simulink model "larix_simulink_gazebo"  (R2020b)
settings: Solver=FixedStepDiscrete  StartTime=0.0  StopTime=inf  RelTol=1e-3  SampleTimeConstraint=Specified
values from neighbouring files (symbols this model uses):
  controller = initController(vehicle, propeller)    [init.m]
  propulsion = initPropulsion()    [init.m]
  sensors = initSensors(vehicle.pos0(3))    [init.m]
  vehicle = initVehicle()    [init.m]
undefined symbols (not defined in the file or in its folder): WMM2020
libraries: robotlib x15, sharedtransform x7, aerolibtransform2 x3, aerolibutil x3, simulink x2, aerolibatmos2 x1, aerolibgravity2 x1
settings Model: PacingRate=0.100000  Creator=pgoldschmid  LastModifiedBy=pgoldschmid

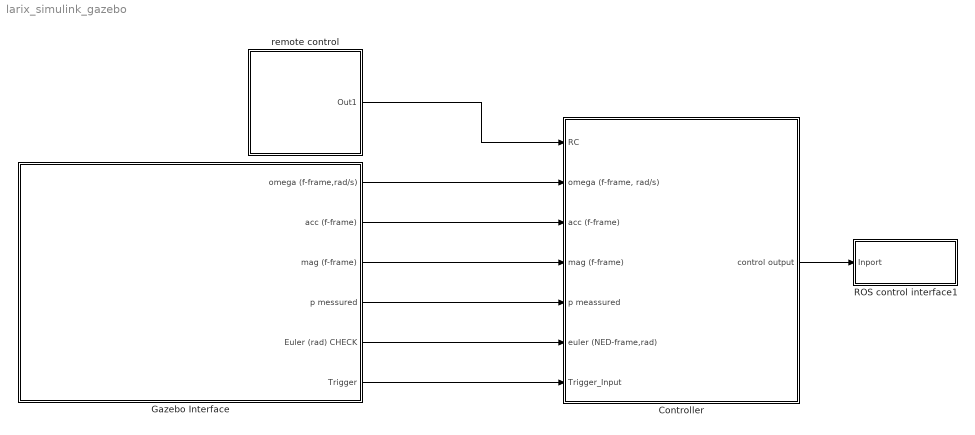
== system larix_simulink_gazebo ==
  Controller : Subsystem
      settings: PortSchema="{\"entries\":[{\"content\":{\"sides\":[{\"content\":{\"connectorIds\":[\"Out1\"]},\"type\":\"ConnectorPlacement.EquallySpacedRectSide\",\"uuid\":\"e6753237-ef8f-4a3a-b26c-e75ae99169a9\"},{\"content\":{\"connectorIds\":[\"In1\",\"In2\",\"In3\",\"In4\",\"In5\",\"In6\",\"In7\"],\"side\":\"RIGHT\"},\"type\":\"ConnectorPlacement.EquallySpacedRectSide\",\"uuid\":\"4f9edf41-85bf-437c-aaf6-18b24e8e6554\"},{\"content\":{\"connectorIds\":[],\"side\":\"TOP\"},\"type\":\"ConnectorPlacement.EquallySpacedRectSide\",\"uuid\":\"a3c7e6d1-df21-4b72-b0cf-f37c3a659b31\"},{\"content\":{\"connectorIds\":[],\"side\":\"BOTTOM\"},\"type\":\"ConnectorPlacement.EquallySpacedRectSide\",\"uuid\":\"23eac58c-75b6-4339-8a58-b1a534739bd3\"},{\"content\":{\"connectorIds\":[],\"side\":\"HIDDEN\"},\"type\":\"ConnectorPlacement.EquallySpacedRectSide\",\"uuid\":\"17e885a9-6a9e-4546-a357-6f7de688dce4\"}]},\"type\":\"ConnectorPlacement.EquallySpacedConnector\",\"uuid\":\"60ad8aaf-2408-428b-b8fd-bb77263ba152\"}],\"packageUris\":[\"http://schema.mathworks.com/mf0/Connector/R2020b\"],\"version\":\"1.0\"}"
  Gazebo Interface : Subsystem  TreatAsAtomicUnit=on
  ROS control interface1 : Subsystem  TreatAsAtomicUnit=on
  remote control : Subsystem  mask{SWA=up, SWB=up, VRA=0.0, VRB=0, SWC=up, SWD=armed (down), ThrustCmd=0.500, YawCmd=0.0, RollCmd=0.0, PitchCmd=0}
      mask prompts: SWA "Switch A"; SWB "Switch B"; VRA "tune 1 (VRA)"; VRB "tune 2 (VRB)"; SWC "Switch C"; SWD "Arming (SW D)"; ThrustCmd "Thrust Command [g]"; YawCmd "Yaw Rate Command [deg/s]"; RollCmd "Roll Command [deg]"; PitchCmd "Pitch Command [deg]"
      mask TypeOptions SWA: up | down
      mask TypeOptions SWB: up | down
      mask TypeOptions SWC: up | center | down
      mask TypeOptions SWD: disarmed (up) | armed (down)
      mask DialogControl ParameterGroupVar Prompt: Simulated Remote Control
      mask Display: image('figures/rc.jpg');
  wires:
  remote control/1(Out1) -> Controller/1(RC)
  Gazebo Interface/1(omega (f-frame,rad/s)) -> Controller/2("omega (f-frame, rad/s)")
  Gazebo Interface/2(acc (f-frame)) -> Controller/3(acc (f-frame))
  Gazebo Interface/3(mag (f-frame)) -> Controller/4(mag (f-frame))
  Gazebo Interface/4(p messured) -> Controller/5(p meassured)
  Gazebo Interface/5(Euler (rad) CHECK) -> Controller/6(euler (NED-frame,rad))
  Controller/1(control output) -> ROS control interface1/1(Inport)
  Gazebo Interface/6(Trigger) -> Controller/7(Trigger_Input)

== system larix_simulink_gazebo/Controller ==
  RC : Inport
  "omega (f-frame, rad/s)" : Inport  Port=2
  acc (f-frame) : Inport  Port=3
  mag (f-frame) : Inport  Port=4
  p meassured : Inport  Port=5
  euler (NED-frame,rad) : Inport  Port=6
  Trigger_Input : Inport  Port=7
  Triggered Subsystem : Subsystem  TreatAsAtomicUnit=on
  control output : Outport  VectorParamsAs1DForOutWhenUnconnected=off
  wires:
  Trigger_Input/1 -> Triggered Subsystem/Trigger
  Triggered Subsystem/1(control output) -> control output/1
  euler (NED-frame,rad)/1 -> Triggered Subsystem/6(euler (NED-frame,rad))
  p meassured/1 -> Triggered Subsystem/5(p meassured)
  mag (f-frame)/1 -> Triggered Subsystem/4(mag (f-frame))
  acc (f-frame)/1 -> Triggered Subsystem/3(acc (f-frame))
  RC/1 -> Triggered Subsystem/1(RC)
  "omega (f-frame, rad/s)"/1 -> Triggered Subsystem/2("omega (f-frame, rad/s)")

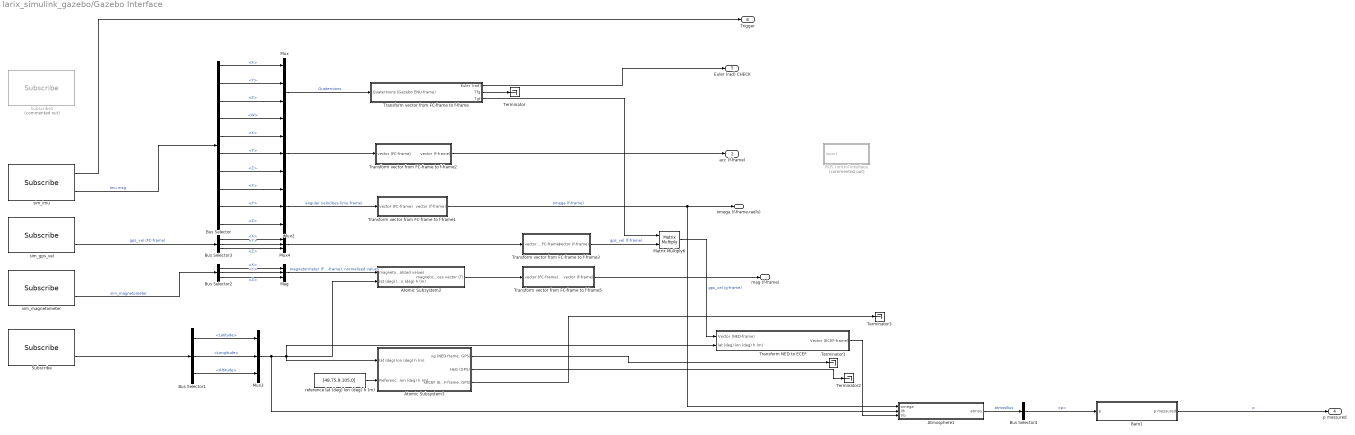
== system larix_simulink_gazebo/Gazebo Interface ==
  " " : Mux  Inputs=3
  Atmosphere1 : Subsystem
  Atomic Subsystem2 : Subsystem  TreatAsAtomicUnit=on
  Atomic Subsystem3 : Subsystem  TreatAsAtomicUnit=on
  Baro1 : Subsystem
  Bus Selector : BusSelector  OutputSignals=Orientation.X,Orientation.Y,Orientation.Z,Orientation.W,LinearAcceleration.X,LinearAcceleration.Y,LinearAcceleration.Z,AngularVelocity.X,AngularVelocity.Y,AngularVelocity.Z
  Bus Selector1 : BusSelector  OutputSignals=Latitude,Longitude,Altitude
  Bus Selector2 : BusSelector  OutputSignals=Vector.X,Vector.Y,Vector.Z
  Bus Selector3 : BusSelector  OutputSignals=Vector.X,Vector.Y,Vector.Z
  Bus Selector4 : BusSelector  OutputSignals=p
  Mag : Mux  Inputs=3
  Matrix Multiply6 : Product  Multiplication=Matrix(*)
  Mux : Mux
  Mux2 : Mux  Inputs=3
  Mux3 : Mux  Inputs=3
  Mux4 : Mux  Inputs=3
  ROS control interface : Subsystem  Commented=on  TreatAsAtomicUnit=on
  Subscribe : robotlib/Subscribe  topicSource=Select from ROS network  topic=/rrbot/sim_gps_fix  messageType=sensor_msgs/NavSatFix  SampleTime=-1  legacyBusStruct=off  messageQueueLength=1
  Subscribe1 : robotlib/Subscribe  Commented=on  topicSource=Select from ROS network  topic=/rrbot/imu_groundtruth  messageType=sensor_msgs/Imu  SampleTime=-1  legacyBusStruct=off  messageQueueLength=1
  Terminator{,1..3} (4 alike) : Terminator
  Transform NED to ECEF : Subsystem  TreatAsAtomicUnit=on
  Transform vector from FC-frame to f-frame : Subsystem  TreatAsAtomicUnit=on
  Transform vector from FC-frame to f-frame1 : Subsystem  TreatAsAtomicUnit=on
  Transform vector from FC-frame to f-frame2 : Subsystem  TreatAsAtomicUnit=on
  Transform vector from FC-frame to f-frame3 : Subsystem  TreatAsAtomicUnit=on
  Transform vector from FC-frame to f-frame5 : Subsystem  TreatAsAtomicUnit=on
  reference lat (deg) lon (deg) h (m) : Constant  Value=[48.75,9.105,0]
  sim_gps_vel : robotlib/Subscribe  topicSource=Select from ROS network  topic=/rrbot/sim_gps_vel  messageType=geometry_msgs/Vector3Stamped  SampleTime=-1  legacyBusStruct=off  messageQueueLength=1
  sim_imu : robotlib/Subscribe  topicSource=Select from ROS network  topic=/rrbot/sim_imu  messageType=sensor_msgs/Imu  SampleTime=-1  legacyBusStruct=off  messageQueueLength=1
  sim_magnetometer : robotlib/Subscribe  topicSource=Select from ROS network  topic=/rrbot/sim_magnetometer  messageType=geometry_msgs/Vector3Stamped  SampleTime=-1  legacyBusStruct=off  messageQueueLength=1
  omega (f-frame,rad/s) : Outport
  acc (f-frame) : Outport  Port=2
  mag (f-frame) : Outport  Port=3
  p messured : Outport  Port=4
  Euler (rad) CHECK : Outport  Port=5
  Trigger : Outport  Port=6
  wires:
  Bus Selector/7 -> " "/3  "<Z>"
  Bus Selector2/1 -> Mag/1  "<X>"
  Mux/1 -> Transform vector from FC-frame to f-frame/1(Quaternions (Gazebo ENU-frame))  "Quaternions"
  Mag/1 -> Atomic Subsystem2/1(magnetometer normalized values)  "magnetormeter (FC-frame), normalized values"
  Atomic Subsystem3/2(" HaG (GPS)") -> Terminator2/1
  Baro1/1(p messured) -> p messured/1  "p"
  Bus Selector/10 -> Mux2/3  "<Z>"
  Bus Selector/6 -> " "/2  "<Y>"
  Bus Selector3/2 -> Mux4/2  "<Y>"
  Bus Selector/8 -> Mux2/1  "<X>"
  Bus Selector4/1 -> Baro1/1(p)  "<p>"
  Transform vector from FC-frame to f-frame/3(Tgf) -> Matrix Multiply6/1
  Transform NED to ECEF/1(Vector (ECEF-frame)) -> Atmosphere1/3(Vb)
  sim_imu/2 -> Bus Selector/1  "Imu msg"
  Bus Selector2/3 -> Mag/3  "<Z>"
  Transform vector from FC-frame to f-frame5/1(vector (f-frame)) -> mag (f-frame)/1
  Bus Selector/3 -> Mux/3  "<Z>"
  Bus Selector2/2 -> Mag/2  "<Y>"
  Matrix Multiply6/1 -> Transform NED to ECEF/1(Vector (NED-frame))  "gps_vel (g-frame)"
  Bus Selector/5 -> " "/1  "<X>"
  Atomic Subsystem2/1(magnetic forces vector (T)) -> Transform vector from FC-frame to f-frame5/1(vector (FC-frame))
  sim_magnetometer/2 -> Bus Selector2/1  "sim_magnetometer"
  Transform vector from FC-frame to f-frame2/1(vector (f-frame)) -> acc (f-frame)/1
  Bus Selector3/3 -> Mux4/3  "<Z>"
  Bus Selector/1 -> Mux/1  "<X>"
  Mux4/1 -> Transform vector from FC-frame to f-frame3/1(vector (FC-frame))
  " "/1 -> Transform vector from FC-frame to f-frame2/1(vector (FC-frame))
  Mux2/1 -> Transform vector from FC-frame to f-frame1/1(vector (FC-frame))  "angular velocities (imu frame)"
  Atomic Subsystem3/1("xg (NED-frame, GPS)") -> Terminator1/1
  Bus Selector/2 -> Mux/2  "<Y>"
  Transform vector from FC-frame to f-frame/1(Euler (rad)) -> Euler (rad) CHECK/1
  Bus Selector/4 -> Mux/4  "<W>"
  Atmosphere1/1(atmos) -> Bus Selector4/1  "atmosBus"
  Bus Selector/9 -> Mux2/2  "<Y>"
  sim_gps_vel/2 -> Bus Selector3/1  "gps_vel (FC-frame)"
  Transform vector from FC-frame to f-frame1/1(vector (f-frame)) -> omega (f-frame,rad/s)/1, Atmosphere1/1(omega)  "omega (f-frame)"
  reference lat (deg) lon (deg) h (m)/1 -> Atomic Subsystem3/2(Reference lat (deg) lon (deg) h (m))
  Bus Selector3/1 -> Mux4/1  "<X>"
  Transform vector from FC-frame to f-frame3/1(vector (f-frame)) -> Matrix Multiply6/2  "gps_vel (f-frame)"
  Atomic Subsystem3/3("xECEF (ECEF-frame, GPS)") -> Terminator3/1
  Mux3/1 -> Atmosphere1/2(llh), Transform NED to ECEF/2(lat (deg) lon (deg) h (m)), Atomic Subsystem2/2(lat (deg) lon (deg) h (m)), Atomic Subsystem3/1(lat (deg) lon (deg) h (m))
  Bus Selector1/1 -> Mux3/1  "<Latitude>"
  Subscribe/2 -> Bus Selector1/1
  Bus Selector1/2 -> Mux3/2  "<Longitude>"
  Bus Selector1/3 -> Mux3/3  "<Altitude>"
  Transform vector from FC-frame to f-frame/2(Tfg) -> Terminator/1
  sim_imu/1 -> Trigger/1

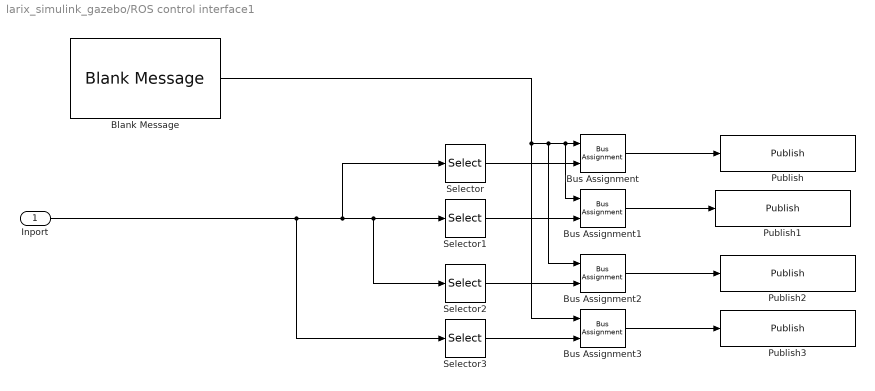
== system larix_simulink_gazebo/ROS control interface1 ==
  Inport : Inport
  Blank Message : robotlib/Blank Message  messageClass=Message  entityType=std_msgs/Float64  messageType=std_msgs/Float64  SampleTime=0.01  legacyBusStruct=off
  Bus Assignment{,1..3} (4 alike) : BusAssignment  AssignedSignals=Data
  Publish : robotlib/Publish  topicSource=Specify your own  topic=/rrbot/simulink_ros_interface/pwm/motor0  messageType=std_msgs/Float64  legacyBusStruct=off  messageQueueLength=1
  Publish1 : robotlib/Publish  topicSource=Specify your own  topic=/rrbot/simulink_ros_interface/pwm/motor1  messageType=std_msgs/Float64  legacyBusStruct=off  messageQueueLength=1
  Publish2 : robotlib/Publish  topicSource=Specify your own  topic=/rrbot/simulink_ros_interface/pwm/motor2  messageType=std_msgs/Float64  legacyBusStruct=off  messageQueueLength=1
  Publish3 : robotlib/Publish  topicSource=Specify your own  topic=/rrbot/simulink_ros_interface/pwm/motor3  messageType=std_msgs/Float64  legacyBusStruct=off  messageQueueLength=1
  Selector : Selector  InputPortWidth=4  IndexOptions=Index vector (dialog)  Indices=1  OutputSizes=1
  Selector1 : Selector  InputPortWidth=4  IndexOptions=Index vector (dialog)  Indices=2  OutputSizes=1
  Selector2 : Selector  InputPortWidth=4  IndexOptions=Index vector (dialog)  Indices=3  OutputSizes=1
  Selector3 : Selector  InputPortWidth=4  IndexOptions=Index vector (dialog)  Indices=4  OutputSizes=1
  wires:
  Inport/1 -> Selector1/1, Selector2/1, Selector/1, Selector3/1
  Selector/1 -> Bus Assignment/2
  Selector2/1 -> Bus Assignment2/2
  Bus Assignment/1 -> Publish/1
  Bus Assignment3/1 -> Publish3/1
  Blank Message/1 -> Bus Assignment/1, Bus Assignment1/1, Bus Assignment2/1, Bus Assignment3/1
  Selector1/1 -> Bus Assignment1/2
  Selector3/1 -> Bus Assignment3/2
  Bus Assignment1/1 -> Publish1/1
  Bus Assignment2/1 -> Publish2/1

== system larix_simulink_gazebo/remote control ==
  note: conversion from [g deg deg deg/s] to PWM
  note: data from mask
  note: example for automatic generation of test signals
  Bias : Bias  Bias=1500
  Bias1 : Bias  Bias=[-1 0 0 0 -1.5 -1.5 0 0 -2 -1.5]
  Bias2 : Bias  Bias=-3
  Demux : Demux  Outputs=10
  Gain : Gain  Gain=[2, 1/45, 1/45, 1/90, 4 4 2 2 2 4]*500
  Mux : Mux  Inputs=10
  Pulse Generator : DiscretePulseGenerator  PulseType=Time based  Amplitude=6  Period=10  PulseWidth=50
  rc : Constant  Value=[ThrustCmd RollCmd PitchCmd YawCmd SWA SWB VRA VRB SWC SWD]
  test signal switch : ManualSwitch
  Out1 : Outport  VectorParamsAs1DForOutWhenUnconnected=off
  wires:
  Demux/10 -> Mux/10
  Demux/9 -> Mux/9
  Demux/8 -> Mux/8
  Demux/7 -> Mux/7
  Demux/6 -> Mux/6
  Demux/5 -> Mux/5
  Demux/2 -> test signal switch/1
  Bias2/1 -> test signal switch/2
  test signal switch/1 -> Mux/2
  Pulse Generator/1 -> Bias2/1
  Mux/1 -> Bias1/1
  rc/1 -> Demux/1
  Demux/4 -> Mux/4
  Demux/3 -> Mux/3
  Demux/1 -> Mux/1
  Bias1/1 -> Gain/1
  Bias/1 -> Out1/1
  Gain/1 -> Bias/1

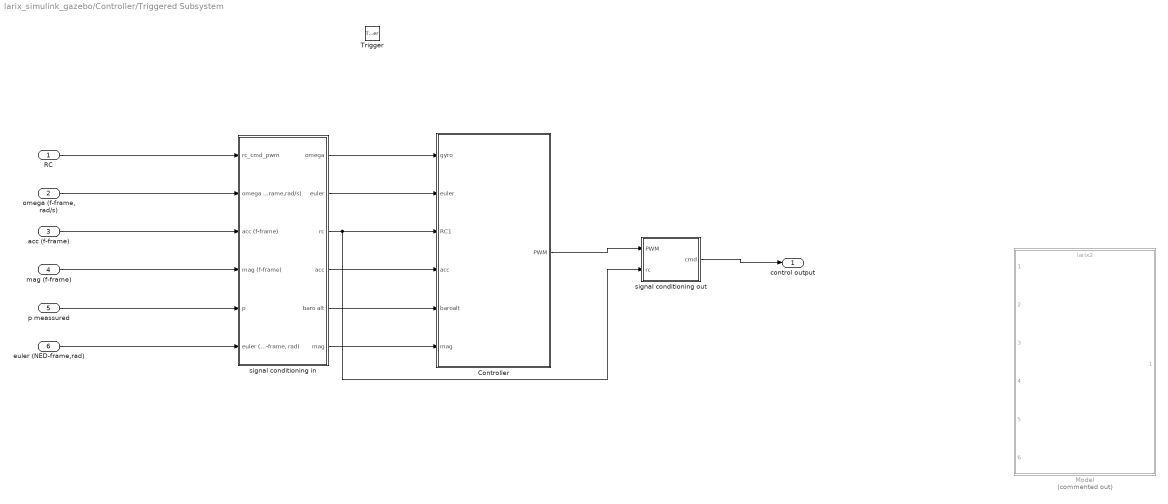
== system larix_simulink_gazebo/Controller/Triggered Subsystem ==
  RC : Inport
  "omega (f-frame, rad/s)" : Inport  Port=2
  acc (f-frame) : Inport  Port=3
  mag (f-frame) : Inport  Port=4
  p meassured : Inport  Port=5
  euler (NED-frame,rad) : Inport  Port=6
  Trigger : TriggerPort  VariantControl=Variant
  Controller : Subsystem  TreatAsAtomicUnit=on
  Model : ModelReference  Commented=on  ModelNameDialog=larix2.slx  SimulationMode=Normal  ModelReferenceVersion=5.6
  signal conditioning in : Subsystem
  signal conditioning out : Subsystem
  control output : Outport
  wires:
  signal conditioning out/1(cmd) -> control output/1
  signal conditioning in/5(baro alt) -> Controller/5(baroalt)
  signal conditioning in/3(rc) -> Controller/3(RC1), signal conditioning out/2(rc)
  signal conditioning in/4(acc) -> Controller/4(acc)
  "omega (f-frame, rad/s)"/1 -> signal conditioning in/2(omega (f-frame,rad/s))
  acc (f-frame)/1 -> signal conditioning in/3(acc (f-frame))
  signal conditioning in/2(euler) -> Controller/2(euler)
  euler (NED-frame,rad)/1 -> signal conditioning in/6("euler (NED-frame, rad)")
  signal conditioning in/1(omega) -> Controller/1(gyro)
  signal conditioning in/6(mag) -> Controller/6(mag)
  RC/1 -> signal conditioning in/1(rc_cmd_pwm)
  mag (f-frame)/1 -> signal conditioning in/4(mag (f-frame))
  p meassured/1 -> signal conditioning in/5(p)
  Controller/1(PWM) -> signal conditioning out/1(PWM)

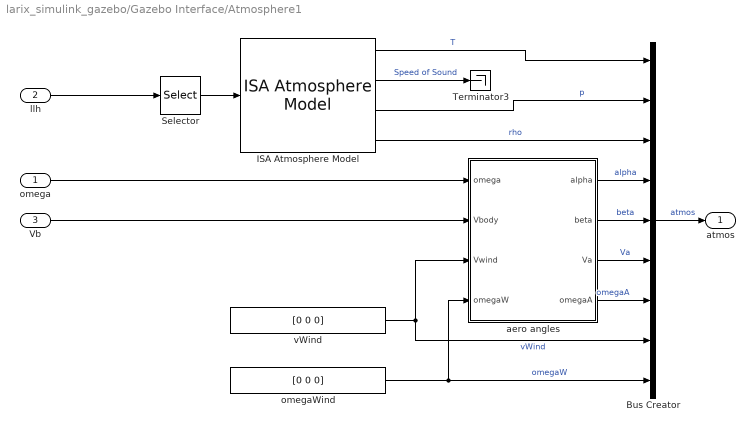
== system larix_simulink_gazebo/Gazebo Interface/Atmosphere1 ==
  omega : Inport
  llh : Inport  Port=2
  Vb : Inport  Port=3
  Bus Creator : BusCreator  Inputs=9
  ISA Atmosphere Model : aerolibatmos2/ISA Atmosphere Model  custom=off  g=9.80665  gamma=1.4  R=287.0531  L=0.0065  h_trop=11000  h_strat=20000  rho0=1.225  P0=101325  T0=288.15  h0=0
  Selector : Selector  InputPortWidth=3  IndexOptions=Index vector (dialog)  Indices=3  OutputSizes=1
  Terminator3 : Terminator
  aero angles : MATLAB Function  TreatAsAtomicUnit=on
  omegaWind : Constant  Value=[0 0 0]  SampleTime=-1
  vWind : Constant  Value=[0 0 0]  SampleTime=-1
  atmos : Outport  VectorParamsAs1DForOutWhenUnconnected=off
  wires:
  vWind/1 -> Bus Creator/8, aero angles/3(Vwind)  "vWind"
  omegaWind/1 -> Bus Creator/9, aero angles/4(omegaW)  "omegaW"
  aero angles/4(omegaA) -> Bus Creator/7  "omegaA"
  Vb/1 -> aero angles/2(Vbody)
  omega/1 -> aero angles/1(omega)
  aero angles/2(beta) -> Bus Creator/5  "beta"
  aero angles/1(alpha) -> Bus Creator/4  "alpha"
  aero angles/3(Va) -> Bus Creator/6  "Va"
  ISA Atmosphere Model/4 -> Bus Creator/3  "rho"
  Selector/1 -> ISA Atmosphere Model/1
  llh/1 -> Selector/1
  ISA Atmosphere Model/2 -> Terminator3/1  "Speed of Sound"
  ISA Atmosphere Model/1 -> Bus Creator/1  "T"
  ISA Atmosphere Model/3 -> Bus Creator/2  "p"
  Bus Creator/1 -> atmos/1  "atmos"

== system larix_simulink_gazebo/Gazebo Interface/Atomic Subsystem2 ==
  magnetometer normalized values : Inport
  lat (deg) lon (deg) h (m) : Inport  Port=2
  Demux : Demux  Outputs=3
  Gain : Gain  Gain=0.000000001
  Product : Product
  World Magnetic Model : aerolibgravity2/World Magnetic Model  model=WMM2020 (2020-2025)  customFile='WMM2020.COF'  units=Metric (MKS)  time_in=off  month=October  day=25  year=2021  action=Error  h_out=off  dec_out=off  inc_out=off  ti_out=on
      settings: SourceProductBaseCode=AE
  magnetic forces vector (T) : Outport
  wires:
  Product/1 -> magnetic forces vector (T)/1
  Gain/1 -> Product/2  "Intensity of magnetic force (T)"
  magnetometer normalized values/1 -> Product/1
  World Magnetic Model/2 -> Gain/1  "Intensity of magnetic force"
  Demux/3 -> World Magnetic Model/1
  Demux/1 -> World Magnetic Model/2
  Demux/2 -> World Magnetic Model/3
  lat (deg) lon (deg) h (m)/1 -> Demux/1

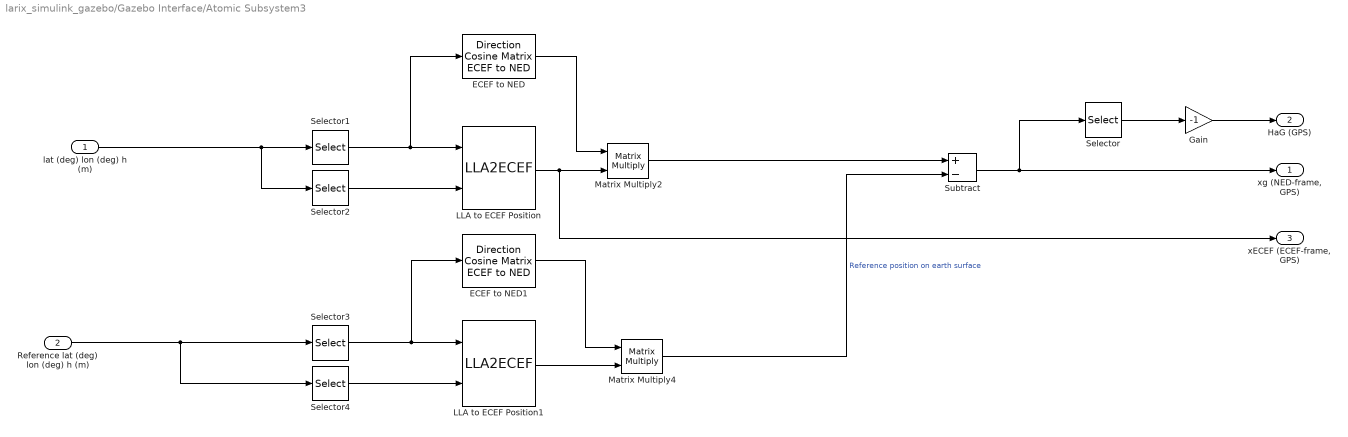
== system larix_simulink_gazebo/Gazebo Interface/Atomic Subsystem3 ==
  lat (deg) lon (deg) h (m) : Inport
  Reference lat (deg) lon (deg) h (m) : Inport  Port=2
  ECEF to NED : aerolibtransform2/Direction Cosine Matrix ECEF to NED
      settings: SourceProductBaseCode=AE
  ECEF to NED1 : aerolibtransform2/Direction Cosine Matrix ECEF to NED
      settings: SourceProductBaseCode=AE
  Gain : Gain  Gain=-1
  LLA to ECEF Position : LLA2ECEF
  LLA to ECEF Position1 : LLA2ECEF
  Matrix Multiply2 : Product  Multiplication=Matrix(*)
  Matrix Multiply4 : Product  Multiplication=Matrix(*)
  Selector : Selector  InputPortWidth=3  IndexOptions=Index vector (dialog)  Indices=[3]  OutputSizes=1
  Selector1 : Selector  InputPortWidth=3  IndexOptions=Index vector (dialog)  Indices=[1 2]  OutputSizes=1
  Selector2 : Selector  InputPortWidth=3  IndexOptions=Index vector (dialog)  Indices=[3]  OutputSizes=1
  Selector3 : Selector  InputPortWidth=3  IndexOptions=Index vector (dialog)  Indices=[1 2]  OutputSizes=1
  Selector4 : Selector  InputPortWidth=3  IndexOptions=Index vector (dialog)  Indices=[3]  OutputSizes=1
  Subtract : Sum  Inputs=+-
  "xg (NED-frame, GPS)" : Outport
  " HaG (GPS)" : Outport  Port=2
  "xECEF (ECEF-frame, GPS)" : Outport  Port=3
  wires:
  ECEF to NED1/1 -> Matrix Multiply4/1
  LLA to ECEF Position1/1 -> Matrix Multiply4/2
  Matrix Multiply4/1 -> Subtract/2  "Reference position on earth surface"
  LLA to ECEF Position/1 -> "xECEF (ECEF-frame, GPS)"/1, Matrix Multiply2/2
  lat (deg) lon (deg) h (m)/1 -> Selector2/1, Selector1/1
  Selector1/1 -> ECEF to NED/1, LLA to ECEF Position/1
  Selector2/1 -> LLA to ECEF Position/2
  ECEF to NED/1 -> Matrix Multiply2/1
  Matrix Multiply2/1 -> Subtract/1
  Reference lat (deg) lon (deg) h (m)/1 -> Selector4/1, Selector3/1
  Selector4/1 -> LLA to ECEF Position1/2
  Selector3/1 -> ECEF to NED1/1, LLA to ECEF Position1/1
  Subtract/1 -> Selector/1, "xg (NED-frame, GPS)"/1
  Selector/1 -> Gain/1
  Gain/1 -> " HaG (GPS)"/1

== system larix_simulink_gazebo/Gazebo Interface/Baro1 ==
  p : Inport  PortDimensions=1
  Baro Bias : Constant  Value=sensors.Baro.Bias
  Baro Noise : RandomNumber  Variance=sensors.Baro.Noise^2
  Manual Switch2 : ManualSwitch
  Sum3 : Sum  Inputs=++|
  Sum4 : Sum  Inputs=++|
  p messured : Outport  PortDimensions=1  VectorParamsAs1DForOutWhenUnconnected=off
  wires:
  Sum3/1 -> Sum4/2
  Sum4/1 -> Manual Switch2/1
  Manual Switch2/1 -> p messured/1
  p/1 -> Manual Switch2/2, Sum3/2  "p [Pa]"
  Baro Bias/1 -> Sum4/1
  Baro Noise/1 -> Sum3/1

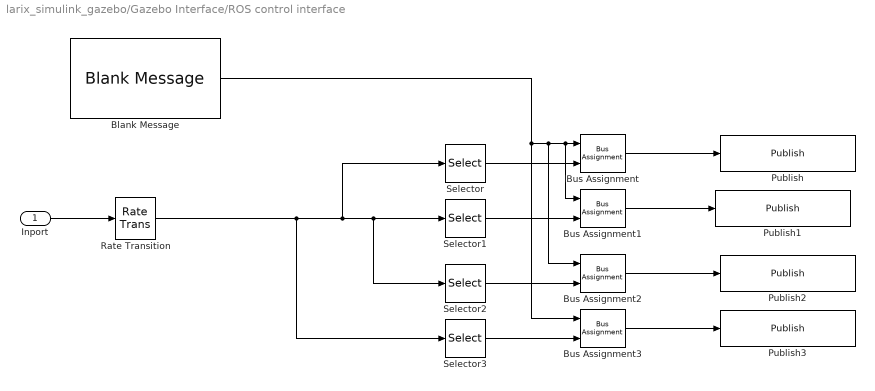
== system larix_simulink_gazebo/Gazebo Interface/ROS control interface ==
  Inport : Inport
  Blank Message : robotlib/Blank Message  messageClass=Message  entityType=std_msgs/Float64  messageType=std_msgs/Float64  SampleTime=0.01  legacyBusStruct=off
  Bus Assignment{,1..3} (4 alike) : BusAssignment  AssignedSignals=Data
  Publish : robotlib/Publish  topicSource=Specify your own  topic=/rrbot/simulink_ros_interface/pwm/motor0  messageType=std_msgs/Float64  legacyBusStruct=off  messageQueueLength=1
  Publish1 : robotlib/Publish  topicSource=Specify your own  topic=/rrbot/simulink_ros_interface/pwm/motor1  messageType=std_msgs/Float64  legacyBusStruct=off  messageQueueLength=1
  Publish2 : robotlib/Publish  topicSource=Specify your own  topic=/rrbot/simulink_ros_interface/pwm/motor2  messageType=std_msgs/Float64  legacyBusStruct=off  messageQueueLength=1
  Publish3 : robotlib/Publish  topicSource=Specify your own  topic=/rrbot/simulink_ros_interface/pwm/motor3  messageType=std_msgs/Float64  legacyBusStruct=off  messageQueueLength=1
  Rate Transition : RateTransition  OutPortSampleTime=0.01
  Selector : Selector  InputPortWidth=4  IndexOptions=Index vector (dialog)  Indices=3  OutputSizes=1
  Selector1 : Selector  InputPortWidth=4  IndexOptions=Index vector (dialog)  Indices=4  OutputSizes=1
  Selector2 : Selector  InputPortWidth=4  IndexOptions=Index vector (dialog)  Indices=2  OutputSizes=1
  Selector3 : Selector  InputPortWidth=4  IndexOptions=Index vector (dialog)  Indices=1  OutputSizes=1
  wires:
  Bus Assignment2/1 -> Publish2/1
  Bus Assignment1/1 -> Publish1/1
  Selector3/1 -> Bus Assignment3/2
  Selector1/1 -> Bus Assignment1/2
  Blank Message/1 -> Bus Assignment3/1, Bus Assignment2/1, Bus Assignment1/1, Bus Assignment/1
  Bus Assignment3/1 -> Publish3/1
  Bus Assignment/1 -> Publish/1
  Selector2/1 -> Bus Assignment2/2
  Selector/1 -> Bus Assignment/2
  Inport/1 -> Rate Transition/1
  Rate Transition/1 -> Selector3/1, Selector/1, Selector2/1, Selector1/1

== system larix_simulink_gazebo/Gazebo Interface/Transform NED to ECEF ==
  Vector (NED-frame) : Inport
  lat (deg) lon (deg) h (m) : Inport  Port=2
  ECEF to NED : aerolibtransform2/Direction Cosine Matrix ECEF to NED
      settings: SourceProductBaseCode=AE
  Matrix Multiply7 : Product  Multiplication=Matrix(*)
  NED to ECEF : aerolibutil/Invert  3x3 Matrix
  Selector1 : Selector  InputPortWidth=3  IndexOptions=Index vector (dialog)  Indices=[1 2]  OutputSizes=1
  Vector (ECEF-frame) : Outport
  wires:
  Selector1/1 -> ECEF to NED/1
  lat (deg) lon (deg) h (m)/1 -> Selector1/1
  NED to ECEF/1 -> Matrix Multiply7/1
  ECEF to NED/1 -> NED to ECEF/1
  Vector (NED-frame)/1 -> Matrix Multiply7/2
  Matrix Multiply7/1 -> Vector (ECEF-frame)/1  "gps_vel (ecef-frame)"

== system larix_simulink_gazebo/Gazebo Interface/Transform vector from FC-frame to f-frame ==
  Quaternions (Gazebo ENU-frame) : Inport
  Quaternions to Tfg : sharedtransform/Quaternions to  Direction Cosine Matrix  aMode=aMode
      settings: SourceProductBaseCode=AE,PW,MT,UV,VE,VP
  Reorder to phi theta psi : Selector  InputPortWidth=3  IndexOptions=Index vector (dialog)  Indices=[3,2,1]  OutputSizes=1
  Rotation angles : sharedtransform/Quaternions to Rotation Angles  rotationOrder=ZYX  aMode=aMode
      settings: SourceProductBaseCode=AE,PW,MT,UV,VE,VP
  Tgf1 : aerolibutil/Invert  3x3 Matrix
  Transform Gazebo ENU-frame to NED-frame : Subsystem  TreatAsAtomicUnit=on
  Euler (rad) : Outport
  Tfg : Outport  Port=2
  Tgf : Outport  Port=3
  wires:
  Reorder to phi theta psi/1 -> Euler (rad)/1
  Quaternions to Tfg/1 -> Tfg/1, Tgf1/1
  Transform Gazebo ENU-frame to NED-frame/1(Quaternion (NED-frame)) -> Rotation angles/1, Quaternions to Tfg/1
  Rotation angles/1 -> Reorder to phi theta psi/1
  Tgf1/1 -> Tgf/1
  Quaternions (Gazebo ENU-frame)/1 -> Transform Gazebo ENU-frame to NED-frame/1("Quaternion (ENU-frame, Gazebo reference)")

== system larix_simulink_gazebo/Gazebo Interface/Transform vector from FC-frame to f-frame1 ==
  vector (FC-frame) : Inport
  Matrix Multiply1 : Product  Multiplication=Matrix(*)
  Rotation angles of FC-frame wrt f-frame : Constant  Value=[3.141592,0,0]
  T_f_FC : sharedtransform/Rotation Angles to Direction Cosine Matrix  rotationOrder=XYZ  aMode=aMode
      settings: SourceProductBaseCode=AE,PW,MT,UV,VE,VP
  vector (f-frame) : Outport
  wires:
  vector (FC-frame)/1 -> Matrix Multiply1/2  "input vector (FC-frame)"
  Matrix Multiply1/1 -> vector (f-frame)/1  "output vector (f-frame)"
  Rotation angles of FC-frame wrt f-frame/1 -> T_f_FC/1
  T_f_FC/1 -> Matrix Multiply1/1

== system larix_simulink_gazebo/Gazebo Interface/Transform vector from FC-frame to f-frame2 ==
  vector (FC-frame) : Inport
  Matrix Multiply1 : Product  Multiplication=Matrix(*)
  Rotation angles of FC-frame wrt f-frame : Constant  Value=[3.141592,0,0]
  T_f_FC : sharedtransform/Rotation Angles to Direction Cosine Matrix  rotationOrder=XYZ  aMode=aMode
      settings: SourceProductBaseCode=AE,PW,MT,UV,VE,VP
  vector (f-frame) : Outport
  wires:
  vector (FC-frame)/1 -> Matrix Multiply1/2  "input vector (FC-frame)"
  Matrix Multiply1/1 -> vector (f-frame)/1  "output vector (f-frame)"
  Rotation angles of FC-frame wrt f-frame/1 -> T_f_FC/1
  T_f_FC/1 -> Matrix Multiply1/1

== system larix_simulink_gazebo/Gazebo Interface/Transform vector from FC-frame to f-frame3 ==
  vector (FC-frame) : Inport
  Matrix Multiply1 : Product  Multiplication=Matrix(*)
  Rotation angles of FC-frame wrt f-frame : Constant  Value=[3.141592,0,0]
  T_f_FC : sharedtransform/Rotation Angles to Direction Cosine Matrix  rotationOrder=XYZ  aMode=aMode
      settings: SourceProductBaseCode=AE,PW,MT,UV,VE,VP
  vector (f-frame) : Outport
  wires:
  vector (FC-frame)/1 -> Matrix Multiply1/2  "input vector (FC-frame)"
  Matrix Multiply1/1 -> vector (f-frame)/1  "output vector (f-frame)"
  Rotation angles of FC-frame wrt f-frame/1 -> T_f_FC/1
  T_f_FC/1 -> Matrix Multiply1/1

== system larix_simulink_gazebo/Gazebo Interface/Transform vector from FC-frame to f-frame5 ==
  vector (FC-frame) : Inport
  Matrix Multiply1 : Product  Multiplication=Matrix(*)
  Rotation angles of FC-frame wrt f-frame : Constant  Value=[3.141592,0,0]
  T_f_FC : sharedtransform/Rotation Angles to Direction Cosine Matrix  rotationOrder=XYZ  aMode=aMode
      settings: SourceProductBaseCode=AE,PW,MT,UV,VE,VP
  vector (f-frame) : Outport
  wires:
  vector (FC-frame)/1 -> Matrix Multiply1/2  "input vector (FC-frame)"
  Matrix Multiply1/1 -> vector (f-frame)/1  "output vector (f-frame)"
  Rotation angles of FC-frame wrt f-frame/1 -> T_f_FC/1
  T_f_FC/1 -> Matrix Multiply1/1

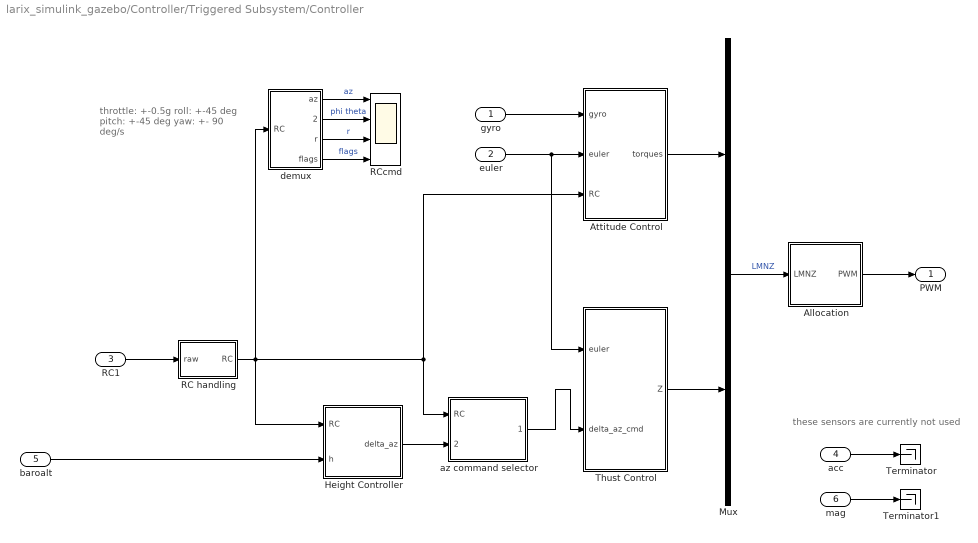
== system larix_simulink_gazebo/Controller/Triggered Subsystem/Controller ==
  note: these sensors are currently not used
  note: throttle: +-0.5g
      | roll: +-45 deg
      | pitch: +-45 deg
      | yaw: +- 90 deg/s
  gyro : Inport  OutDataTypeStr=single  PortDimensions=3
  euler : Inport  Port=2  OutDataTypeStr=single  PortDimensions=3
  RC1 : Inport  Port=3  OutDataTypeStr=single  PortDimensions=10
  acc : Inport  Port=4  OutDataTypeStr=single  PortDimensions=3
  baroalt : Inport  Port=5  OutDataTypeStr=single  PortDimensions=1
  mag : Inport  Port=6  OutDataTypeStr=single  PortDimensions=3
  Allocation : Subsystem
  Attitude Control : Subsystem
  Height Controller : Subsystem
  Mux : Mux  Inputs=2
  RC handling : Subsystem
  RCcmd : Scope  NumInputPorts=4
  Terminator : Terminator
  Terminator1 : Terminator
  Thust Control : Subsystem
  az command selector : Subsystem
  demux : Subsystem
  PWM : Outport  OutDataTypeStr=single  PortDimensions=4  VectorParamsAs1DForOutWhenUnconnected=off
  wires:
  Height Controller/1(delta_az) -> az command selector/2(az_hctrl)
  RC1/1 -> RC handling/1(raw)
  Mux/1 -> Allocation/1(LMNZ)  "LMNZ"
  mag/1 -> Terminator1/1
  demux/3(r) -> RCcmd/3  "r"
  demux/1(az) -> RCcmd/1  "az"
  az command selector/1(az_cmd) -> Thust Control/2(delta_az_cmd)
  Attitude Control/1(torques) -> Mux/1
  baroalt/1 -> Height Controller/2(h)
  demux/2(phitheta) -> RCcmd/2  "phi theta"
  acc/1 -> Terminator/1
  demux/4(flags) -> RCcmd/4  "flags"
  euler/1 -> Thust Control/1(euler), Attitude Control/2(euler)
  Thust Control/1(Z) -> Mux/2
  gyro/1 -> Attitude Control/1(gyro)
  RC handling/1(RC) -> az command selector/1(RC), Attitude Control/3(RC), Height Controller/1(RC), demux/1(RC)
  Allocation/1(PWM) -> PWM/1

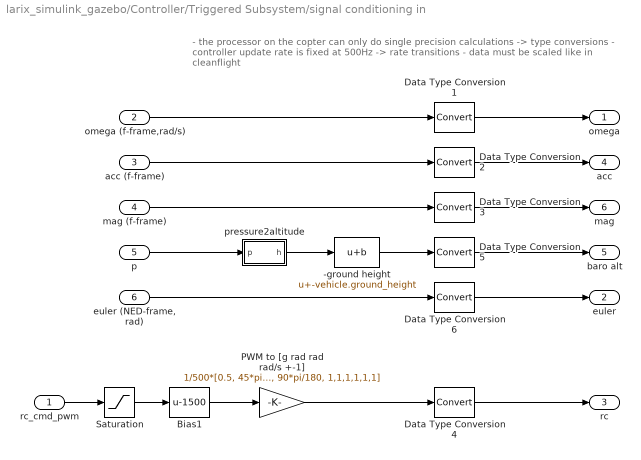
== system larix_simulink_gazebo/Controller/Triggered Subsystem/signal conditioning in ==
  note: - the processor on the copter can only do single precision calculations -> type conversions
      | - controller update rate is fixed at 500Hz -> rate transitions
      | - data must be scaled like in cleanflight
  rc_cmd_pwm : Inport  PortDimensions=10
  omega (f-frame,rad/s) : Inport  Port=2
  acc (f-frame) : Inport  Port=3
  mag (f-frame) : Inport  Port=4
  p : Inport  Port=5
  "euler (NED-frame, rad)" : Inport  Port=6
  -ground height : Bias  Bias=-vehicle.ground_height
  Bias1 : Bias  Bias=-1500
  Data Type Conversion{1..6} (6 alike) : DataTypeConversion
  PWM to [g rad rad rad/s +-1] : Gain  Gain=1/500*[0.5, 45*pi/180, 45*pi/180, 90*pi/180, 1,1,1,1,1,1]
  Saturation : Saturate  UpperLimit=2000  LowerLimit=1000
  pressure2altitude : MATLAB Function  TreatAsAtomicUnit=on
  omega : Outport  VectorParamsAs1DForOutWhenUnconnected=off
  euler : Outport  Port=2  PortDimensions=3  VectorParamsAs1DForOutWhenUnconnected=off
  rc : Outport  Port=3  VectorParamsAs1DForOutWhenUnconnected=off
  acc : Outport  Port=4  VectorParamsAs1DForOutWhenUnconnected=off
  baro alt : Outport  Port=5  VectorParamsAs1DForOutWhenUnconnected=off
  mag : Outport  Port=6  VectorParamsAs1DForOutWhenUnconnected=off
  wires:
  "euler (NED-frame, rad)"/1 -> Data Type Conversion6/1
  omega (f-frame,rad/s)/1 -> Data Type Conversion1/1
  PWM to [g rad rad rad/s +-1]/1 -> Data Type Conversion4/1
  Bias1/1 -> PWM to [g rad rad rad/s +-1]/1
  Data Type Conversion6/1 -> euler/1
  Saturation/1 -> Bias1/1
  rc_cmd_pwm/1 -> Saturation/1
  Data Type Conversion4/1 -> rc/1
  Data Type Conversion5/1 -> baro alt/1
  Data Type Conversion3/1 -> mag/1
  Data Type Conversion2/1 -> acc/1
  Data Type Conversion1/1 -> omega/1
  mag (f-frame)/1 -> Data Type Conversion3/1
  acc (f-frame)/1 -> Data Type Conversion2/1
  p/1 -> pressure2altitude/1(p)
  -ground height/1 -> Data Type Conversion5/1
  pressure2altitude/1(h) -> -ground height/1

== system larix_simulink_gazebo/Controller/Triggered Subsystem/signal conditioning out ==
  note: this simulates the arming handling
      | inside the onboard computer
      | (engines off if switch off)
  PWM : Inport
  rc : Inport  Port=2
  Compare To Constant : simulink/Logic and Bit Operations/Compare To Constant  relop=>  const=0  OutDataTypeStr=boolean
  Data Type Conversion1 : DataTypeConversion
  Delay2 : Delay  DelayLength=1
  Selector : Selector  IndexMode=Zero-based  InputPortWidth=10  IndexOptions=Index vector (dialog)  Indices=9  OutputSizes=1
  Switch : Switch  Criteria=u2 > Threshold
  motors off : Constant  Value=1000.*ones(4,1)
  cmd : Outport  VectorParamsAs1DForOutWhenUnconnected=off
  wires:
  rc/1 -> Selector/1
  motors off/1 -> Switch/3
  Delay2/1 -> Switch/1
  Switch/1 -> cmd/1
  Compare To Constant/1 -> Switch/2
  Selector/1 -> Compare To Constant/1
  Data Type Conversion1/1 -> Delay2/1
  PWM/1 -> Data Type Conversion1/1

== system larix_simulink_gazebo/Gazebo Interface/Transform vector from FC-frame to f-frame/Transform Gazebo ENU-frame to NED-frame ==
  "Quaternion (ENU-frame, Gazebo reference)" : Inport
  Constant : Constant  Value=[0,0,pi/2]
  Gain : Gain  Gain=[1,1,-1,-1]
  Quaternion Multiplication : aerolibutil/Quaternion Multiplication
  Reorder real part : Selector  InputPortWidth=4  IndexOptions=Index vector (dialog)  Indices=[4,1,2,3]  OutputSizes=1
  Rotation Angles to Quaternions : sharedtransform/Rotation Angles to Quaternions  rotationOrder=XYZ  aMode=aMode
      settings: SourceProductBaseCode=AE,PW,MT,UV,VE,VP
  Quaternion (NED-frame) : Outport
  wires:
  "Quaternion (ENU-frame, Gazebo reference)"/1 -> Reorder real part/1
  Quaternion Multiplication/1 -> Quaternion (NED-frame)/1
  Constant/1 -> Rotation Angles to Quaternions/1
  Rotation Angles to Quaternions/1 -> Quaternion Multiplication/1
  Reorder real part/1 -> Gain/1
  Gain/1 -> Quaternion Multiplication/2

== system larix_simulink_gazebo/Controller/Triggered Subsystem/Controller/Allocation ==
  note: We get torques and a force from the controllers and need to distribute these commands among the motors.
      | In addition we need to convert these values into commands the ESCs can understand
  LMNZ : Inport
  1-D Lookup Table1 : Lookup_n-D  NumberOfTableDimensions=1  BreakpointsForDimension1=propulsion.thrust  BreakpointsForDimension1DataTypeStr=single  Table=propulsion.PWM  TableDataTypeStr=single  IntermediateResultsDataTypeStr=single  RemoveProtectionInput=on  InternalRulePriority=Speed  OutDataTypeStr=single  RndMeth=Simplest  FractionDataTypeStr=single  InputSameDT=on
  Allocation : Gain  Gain=controller.allocation  Multiplication=Matrix(K*u)  ParamDataTypeStr=single
  Saturation : Saturate  UpperLimit=1600  LowerLimit=1150  OutDataTypeStr=single
  controller output : Scope  NumInputPorts=3
  PWM : Outport  VectorParamsAs1DForOutWhenUnconnected=off
  wires:
  Saturation/1 -> PWM/1
  LMNZ/1 -> Allocation/1, controller output/1  "LMNZ"
  1-D Lookup Table1/1 -> controller output/3, Saturation/1  "PWM [1000-2000]"
  Allocation/1 -> controller output/2, 1-D Lookup Table1/1  "individual thrusts"

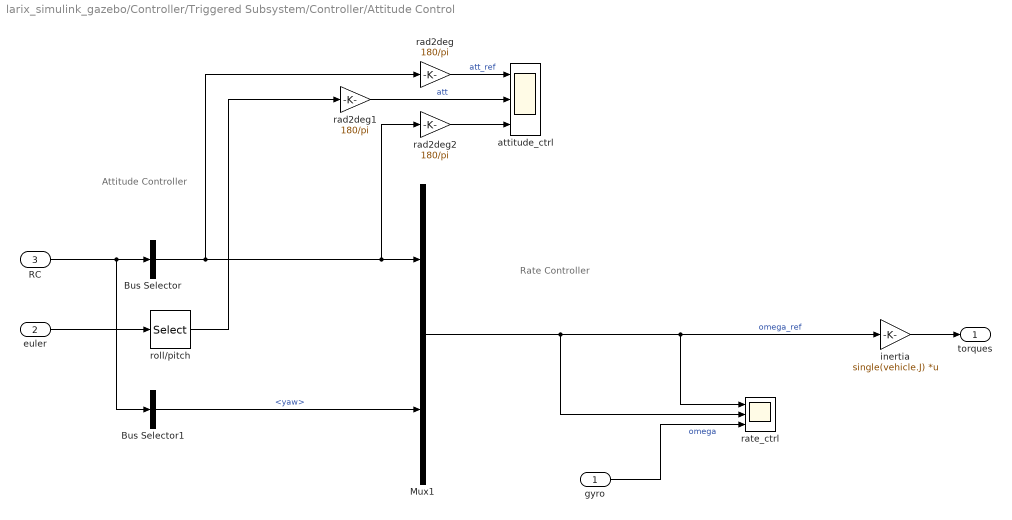
== system larix_simulink_gazebo/Controller/Triggered Subsystem/Controller/Attitude Control ==
  note: Rate Controller
  note: Attitude Controller
  gyro : Inport  OutDataTypeStr=single  PortDimensions=3
  euler : Inport  Port=2
  RC : Inport  Port=3
  Bus Selector : BusSelector  OutputSignals=TRPY.roll,TRPY.pitch  OutputAsBus=on
  Bus Selector1 : BusSelector  OutputSignals=TRPY.yaw
  Mux1 : Mux  Inputs=2
  attitude_ctrl : Scope  NumInputPorts=3
  inertia : Gain  Gain=single(vehicle.J)  Multiplication=Matrix(K*u)  ParamDataTypeStr=single
  rad2deg : Gain  Gain=180/pi
  rad2deg1 : Gain  Gain=180/pi
  rad2deg2 : Gain  Gain=180/pi
  rate_ctrl : Scope  NumInputPorts=3
  roll/pitch : Selector  IndexMode=Zero-based  InputPortWidth=3  IndexOptions=Index vector (dialog)  Indices=[0 1]  OutputSizes=1
  torques : Outport  VectorParamsAs1DForOutWhenUnconnected=off
  wires:
  roll/pitch/1 -> rad2deg1/1
  euler/1 -> roll/pitch/1
  RC/1 -> Bus Selector1/1, Bus Selector/1
  Mux1/1 -> inertia/1, rate_ctrl/1, rate_ctrl/2  "omega_ref"
  gyro/1 -> rate_ctrl/3  "omega"
  inertia/1 -> torques/1
  rad2deg/1 -> attitude_ctrl/1  "att_ref"
  rad2deg1/1 -> attitude_ctrl/2  "att"
  rad2deg2/1 -> attitude_ctrl/3
  Bus Selector1/1 -> Mux1/2  "<yaw>"
  Bus Selector/1 -> rad2deg/1, rad2deg2/1, Mux1/1

== system larix_simulink_gazebo/Controller/Triggered Subsystem/Controller/Height Controller ==
  RC : Inport
  h : Inport  Port=2  OutDataTypeStr=single  PortDimensions=1
  Bus Selector : BusSelector  OutputSignals=TRPY,armed
  Height Reference : Subsystem
  Mux : Mux  Inputs=2
  Saturation : Saturate  UpperLimit=100  LowerLimit=0
  height controller : Scope
  delta_az : Outport  OutDataTypeStr=single  PortDimensions=1  VectorParamsAs1DForOutWhenUnconnected=off
  wires:
  h/1 -> Height Reference/3(h), Mux/2  "h"
  Saturation/1 -> delta_az/1, Mux/1  "a_cmd"
  Mux/1 -> height controller/1  "h"
  Height Reference/1(h_ref) -> Saturation/1
  Bus Selector/1 -> Height Reference/1(RC)  "<TRPY>"
  Bus Selector/2 -> Height Reference/2(armed)  "<armed>"
  RC/1 -> Bus Selector/1

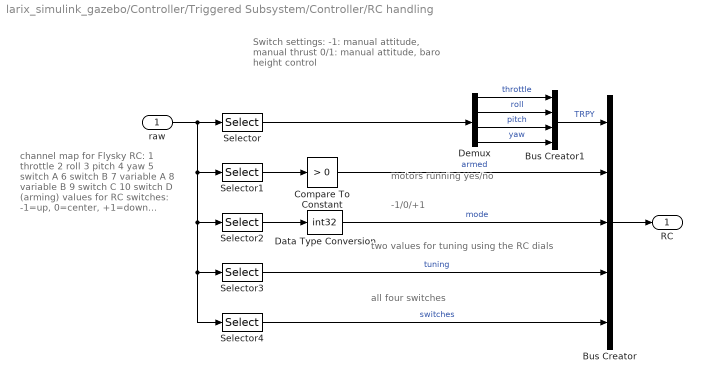
== system larix_simulink_gazebo/Controller/Triggered Subsystem/Controller/RC handling ==
  note: all four switches
  note: two values for tuning using the RC dials
  note: motors running yes/no
  note: channel map for Flysky RC:
      | 1 throttle
      | 2 roll
      | 3 pitch
      | 4 yaw
      | 5 switch A
      | 6 switch B
      | 7 variable A
      | 8 variable B
      | 9 switch C
      | 10 switch D (arming)
      |
      | values for RC switches:
      |      -1=up, 0=center, +1=down
      |     (-1/+1 for 2 position switches)
  note: -1/0/+1
  note: Switch settings:
      | -1: manual attitude, manual thrust
      | 0/1: manual attitude, baro height control
  raw : Inport
  Bus Creator : BusCreator  Inputs=5
  Bus Creator1 : BusCreator  Inputs=4
  Compare To Constant : simulink/Logic and Bit Operations/Compare To Constant  relop=>  const=0  OutDataTypeStr=boolean
  Data Type Conversion : DataTypeConversion  OutDataTypeStr=int32
  Demux : Demux
  Selector : Selector  IndexMode=Zero-based  InputPortWidth=10  IndexOptions=Index vector (dialog)  Indices=0:3  OutputSizes=1
  Selector1 : Selector  IndexMode=Zero-based  InputPortWidth=10  IndexOptions=Index vector (dialog)  Indices=9  OutputSizes=1
  Selector2 : Selector  IndexMode=Zero-based  InputPortWidth=10  IndexOptions=Index vector (dialog)  Indices=8  OutputSizes=1
  Selector3 : Selector  IndexMode=Zero-based  InputPortWidth=10  IndexOptions=Index vector (dialog)  Indices=6:7  OutputSizes=1
  Selector4 : Selector  IndexMode=Zero-based  InputPortWidth=10  IndexOptions=Index vector (dialog)  Indices=[4,5,8,9]  OutputSizes=1
  RC : Outport  VectorParamsAs1DForOutWhenUnconnected=off
  wires:
  raw/1 -> Selector4/1, Selector3/1, Selector2/1, Selector1/1, Selector/1
  Bus Creator1/1 -> Bus Creator/1  "TRPY"
  Selector2/1 -> Data Type Conversion/1
  Selector1/1 -> Compare To Constant/1
  Compare To Constant/1 -> Bus Creator/2  "armed"
  Data Type Conversion/1 -> Bus Creator/3  "mode"
  Selector3/1 -> Bus Creator/4  "tuning"
  Bus Creator/1 -> RC/1
  Selector4/1 -> Bus Creator/5  "switches"
  Demux/1 -> Bus Creator1/1  "throttle"
  Demux/2 -> Bus Creator1/2  "roll"
  Demux/3 -> Bus Creator1/3  "pitch"
  Demux/4 -> Bus Creator1/4  "yaw"
  Selector/1 -> Demux/1

== system larix_simulink_gazebo/Controller/Triggered Subsystem/Controller/Thust Control ==
  euler : Inport  OutDataTypeStr=single  PortDimensions=3
  delta_az_cmd : Inport  Port=2  OutDataTypeStr=single  PortDimensions=1
  Product : Product
  Saturation2 : Saturate  UpperLimit=0.05
  g : Gain  Gain=single(9.806)
  hover offset : Bias  Bias=1
  mass : Gain  Gain=single(vehicle.m)  ParamDataTypeStr=single
  tilt compensation : Subsystem
  Z : Outport  OutDataTypeStr=single  PortDimensions=1  VectorParamsAs1DForOutWhenUnconnected=off
  wires:
  hover offset/1 -> g/1  "0.5-1.5g"
  mass/1 -> Z/1  "Z"
  delta_az_cmd/1 -> Saturation2/1
  Saturation2/1 -> Product/2  "+-0.5g delta_a"
  g/1 -> mass/1
  tilt compensation/1(az_multiplier) -> Product/1
  euler/1 -> tilt compensation/1(euler)
  Product/1 -> hover offset/1

== system larix_simulink_gazebo/Controller/Triggered Subsystem/Controller/az command selector ==
  note: depending on the mode, we either use the acceleration command
      | from the height controller or directly from the RC
  RC : Inport
  az_hctrl : Inport  Port=2
  Bus Selector : BusSelector  OutputSignals=mode
  Bus Selector1 : BusSelector  OutputSignals=TRPY.throttle
  az_cmd_selector : MultiPortSwitch  DataPortOrder=Specify indices  DataPortIndices={[0,1],[-1]}
  az_cmd : Outport  VectorParamsAs1DForOutWhenUnconnected=off
  wires:
  RC/1 -> Bus Selector1/1, Bus Selector/1
  Bus Selector1/1 -> az_cmd_selector/3  "<throttle>"
  az_cmd_selector/1 -> az_cmd/1
  Bus Selector/1 -> az_cmd_selector/1  "<mode>"
  az_hctrl/1 -> az_cmd_selector/2

== system larix_simulink_gazebo/Controller/Triggered Subsystem/Controller/demux ==
  RC : Inport
  Bus Selector : BusSelector  OutputSignals=TRPY,armed,mode
  Data Type Conversion : DataTypeConversion  OutDataTypeStr=int32
  Demux : Demux
  Mux1 : Mux  Inputs=2
  Mux2 : Mux  Inputs=2
  rad2deg : Gain  Gain=single([1, 180/pi, 180/pi, 180/pi])  ParamDataTypeStr=single
  az : Outport  VectorParamsAs1DForOutWhenUnconnected=off
  phitheta : Outport  Port=2  VectorParamsAs1DForOutWhenUnconnected=off
  r : Outport  Port=3  VectorParamsAs1DForOutWhenUnconnected=off
  flags : Outport  Port=4  VectorParamsAs1DForOutWhenUnconnected=off
  wires:
  Demux/1 -> az/1  "az"
  Demux/4 -> r/1  "r"
  rad2deg/1 -> Demux/1
  Demux/3 -> Mux1/2
  Demux/2 -> Mux1/1
  Mux1/1 -> phitheta/1
  Bus Selector/2 -> Data Type Conversion/1  "<armed>"
  Bus Selector/3 -> Mux2/2  "<mode>"
  Mux2/1 -> flags/1
  Data Type Conversion/1 -> Mux2/1
  RC/1 -> Bus Selector/1
  Bus Selector/1 -> rad2deg/1  "<TRPY>"

== system larix_simulink_gazebo/Controller/Triggered Subsystem/Controller/Height Controller/Height Reference ==
  note: Integriert ein von der Fernsteuerung kommendes h_punkt zu einer Sollhöhe auf.
      | Integration wird gestoppt, wenn der Höhenregler abgeschaltet ist (switch=1).
      | Totbereich, damit die Sollhöhe bei zentriertem Stick konstant bleibt.
      | Beim Einschalten wird die aktuelle Höhe als Anfangwert für die Integration übernommen.
  RC : Inport  PortDimensions=4
  armed : Inport  Port=2
  h : Inport  Port=3  PortDimensions=1
  Dead Zone : DeadZone  LowerValue=-0.1  UpperValue=0.1  SaturateOnIntegerOverflow=on
  Logical Operator : Logic  Operator=NOT  AllPortsSameDT=off  OutDataTypeStr=boolean
  Saturation2 : Saturate  OutDataTypeStr=single
  TriggeredIntegrator : Subsystem  TreatAsAtomicUnit=on
  thrust : Selector  IndexMode=Zero-based  InputPortWidth=4  IndexOptions=Index vector (dialog)  Indices=0  OutputSizes=1
  h_ref : Outport  VectorParamsAs1DForOutWhenUnconnected=off
  wires:
  RC/1 -> thrust/1
  Saturation2/1 -> Dead Zone/1
  TriggeredIntegrator/1(y) -> h_ref/1
  thrust/1 -> Saturation2/1
  Logical Operator/1 -> TriggeredIntegrator/2(Enabled)  "disable integration"
  Dead Zone/1 -> TriggeredIntegrator/1(dx)  "h_dot"
  h/1 -> TriggeredIntegrator/3(x0)
  armed/1 -> Logical Operator/1

== system larix_simulink_gazebo/Controller/Triggered Subsystem/Controller/Thust Control/tilt compensation ==
  note: tilted thrust: hdd = F_z * cos(phi)*cos(theta)
      | --> compensation function: 1/(cos(phi)*cos(tehta))
  euler : Inport
  Math Function : Math  Operator=reciprocal  SignedPower=on  OutDataTypeStr=single  SaturateOnIntegerOverflow=on
  Product of Elements : Product  Inputs=*  OutDataTypeStr=single
  Saturation : Saturate  UpperLimit=1.3  LowerLimit=1
  Saturation1 : Saturate  UpperLimit=45*pi/180  LowerLimit=-45*pi/180
  Selector : Selector  IndexMode=Zero-based  InputPortWidth=3  IndexOptions=Index vector (dialog)  Indices=[0 1]  OutputSizes=1
  Trigonometric Function : Trigonometry  Operator=cos  OutputSignalType=real
  az_multiplier : Outport  VectorParamsAs1DForOutWhenUnconnected=off
  wires:
  euler/1 -> Selector/1
  Selector/1 -> Saturation1/1
  Saturation/1 -> az_multiplier/1
  Math Function/1 -> Saturation/1
  Trigonometric Function/1 -> Product of Elements/1
  Product of Elements/1 -> Math Function/1
  Saturation1/1 -> Trigonometric Function/1

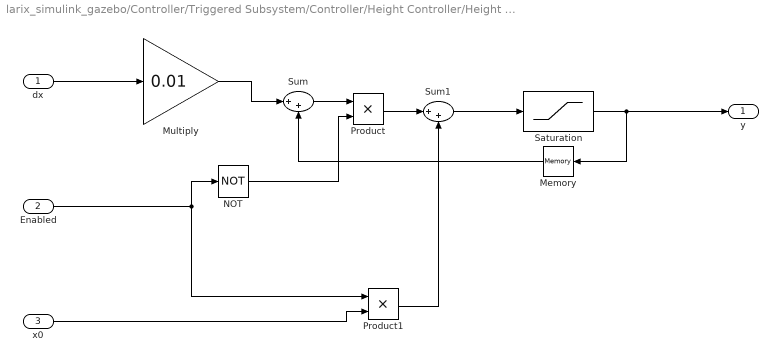
== system larix_simulink_gazebo/Controller/Triggered Subsystem/Controller/Height Controller/Height Reference/TriggeredIntegrator ==
  dx : Inport
  Enabled : Inport  Port=2
  x0 : Inport  Port=3
  Memory : Memory  InheritSampleTime=on
  Multiply : Gain  Gain=0.01  OutDataTypeStr=Inherit: Same as input
  NOT : Logic  Operator=NOT  IconShape=distinctive  AllPortsSameDT=off  OutDataTypeStr=boolean
  Product : Product
  Product1 : Product
  Saturation : Saturate  UpperLimit=50  LowerLimit=-2
  Sum : Sum  Inputs=|++
  Sum1 : Sum  Inputs=|++
  y : Outport
  wires:
  Multiply/1 -> Sum/1
  Memory/1 -> Sum/2
  Saturation/1 -> y/1, Memory/1
  Sum/1 -> Product/1
  dx/1 -> Multiply/1
  Enabled/1 -> NOT/1, Product1/1
  Product1/1 -> Sum1/2
  NOT/1 -> Product/2
  Product/1 -> Sum1/1
  Sum1/1 -> Saturation/1
  x0/1 -> Product1/2

== matlab function larix_simulink_gazebo/Controller/Triggered Subsystem/signal conditioning in/pressure2altitude ==
  data: p input; h output
function h = fcn(p)

h = (288.15/0.0065) * (1 - (p/101325) ^ (1/5.255));


end

== matlab function larix_simulink_gazebo/Gazebo Interface/Atmosphere1/aero angles ==
  data: omega input size=3; Vbody input; Vwind input; omegaW input size=3; alpha output; beta output; Va output; omegaA output size=3
function [alpha,beta,Va,omegaA] = calcAeroAngles(omega,Vbody,Vwind,omegaW)

bVa = Vbody + Vwind;
Va    = norm(bVa);
omegaA = omega + omegaW;

if abs(bVa(1))>1
    alpha = atan2(bVa(3),bVa(1));
else
    alpha = 0;
end

if norm(bVa)>1
    beta  = asin(bVa(2)/norm(bVa));
else
    beta = 0;
end

end
